simulink model "Sim_Modell_v5"  (R2021b)
settings: Solver=daessc  StartTime=0.0  StopTime=100  RelTol=1e-3
undefined symbols (not defined in the file): neg, pos, sigbuilder_block
libraries: fl_lib x25, nesl_utility x17, ee_lib x1, simulink x1
settings Model: Creator=lisa-  LastModifiedBy=felix

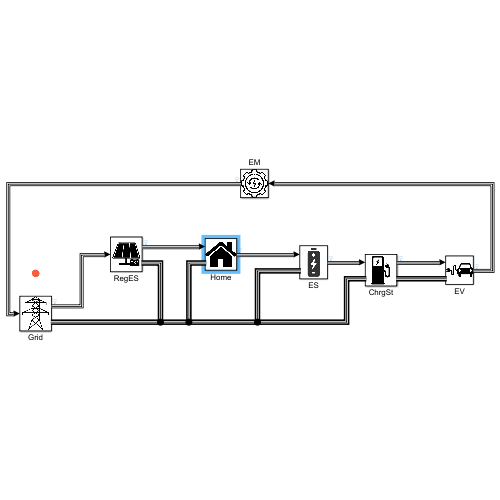
[thumbnail: Simulink's stored preview of the top-level diagram]
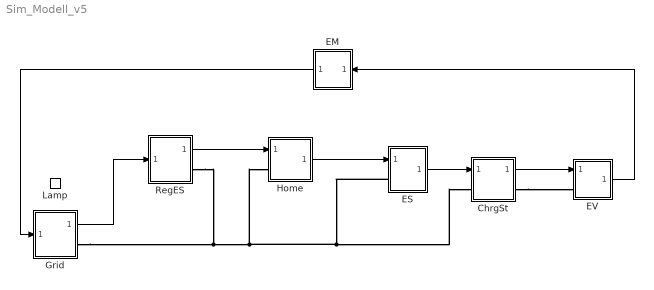
== system Sim_Modell_v5 ==
  ChrgSt : Subsystem
      settings: PortSchema="{\"entries\":[{\"content\":{\"sides\":[{\"content\":{\"connectorIds\":[]},\"type\":\"ConnectorPlacement.EquallySpacedRectSide\",\"uuid\":\"b41e38a9-5af4-4fc3-8362-b0a2c9ea7f09\"},{\"content\":{\"connectorIds\":[],\"side\":\"RIGHT\"},\"type\":\"ConnectorPlacement.EquallySpacedRectSide\",\"uuid\":\"3d2284f1-ff92-4301-996c-df10035f8991\"},{\"content\":{\"connectorIds\":[\"In1\",\"LConn1\"],\"side\":\"TOP\"},\"type\":\"ConnectorPlacement.EquallySpacedRectSide\",\"uuid\":\"3c162699-1ee7-4b12-b844-90d345f681c2\"},{\"content\":{\"connectorIds\":[\"Out1\",\"RConn1\"],\"side\":\"BOTTOM\"},\"type\":\"ConnectorPlacement.EquallySpacedRectSide\",\"uuid\":\"c143c3a3-5e1b-42e8-ba00-2d87f1345ae6\"}]},\"type\":\"ConnectorPlacement.EquallySpacedConnector\",\"uuid\":\"20a307e0-46b7-49be-a325-e97621053049\"}],\"packageUris\":[\"http://schema.mathworks.com/mf0/Connector/R2020b\"],\"version\":\"1.0\"}"
      mask Display: image('D:\Felix\Studium HTW Dresden\8. Semester\Matlab\Bilder\ChrgSt_icon.png'); % Use "Edit Image" on toolstrip to change.
  EM : Subsystem
      mask Display: image('D:\Felix\Studium HTW Dresden\8. Semester\Matlab\Bilder\EM_icon.png'); % Use "Edit Image" on toolstrip to change.
  ES : Subsystem
      mask Display: image('D:\Felix\Studium HTW Dresden\8. Semester\Matlab\Bilder\ES_icon.png'); % Use "Edit Image" on toolstrip to change.
  EV : Subsystem
      mask Display: image('D:\Felix\Studium HTW Dresden\8. Semester\Matlab\Bilder\electric_car_icon.jpg'); % Use "Edit Image" on toolstrip to change.
  Grid : Subsystem
      mask Display: image('D:\Felix\Studium HTW Dresden\8. Semester\Matlab\Bilder\Grid_icon.webp'); % Use "Edit Image" on toolstrip to change.
  Home : Subsystem
      mask Display: image('D:\Felix\Studium HTW Dresden\8. Semester\Matlab\Bilder\Home_icon.png'); % Use "Edit Image" on toolstrip to change.
  Lamp : LampBlock  LabelPosition=Hide
  RegES : Subsystem
      mask Display: image('D:\Felix\Studium HTW Dresden\8. Semester\Matlab\Bilder\solar_storage_icon.png'); % Use "Edit Image" on toolstrip to change.
  wires:
  RegES/1(Out1) -> Home/1(In1)
  Grid/1(Out1) -> RegES/1(In1)
  ES/1(Out1) -> ChrgSt/1(In1)
  ChrgSt/1(Out1) -> EV/1(In1)
  EV/1(Out1) -> EM/1(In1)
  Home/1(Out1) -> ES/1(In1)
  EM/1(Out1) -> Grid/1(In1)
  connections:
  Grid/RConn1 -- RegES/RConn1 -- ES/LConn1 -- ChrgSt/LConn1 -- Home/LConn1
  ChrgSt/RConn1 -- EV/LConn1

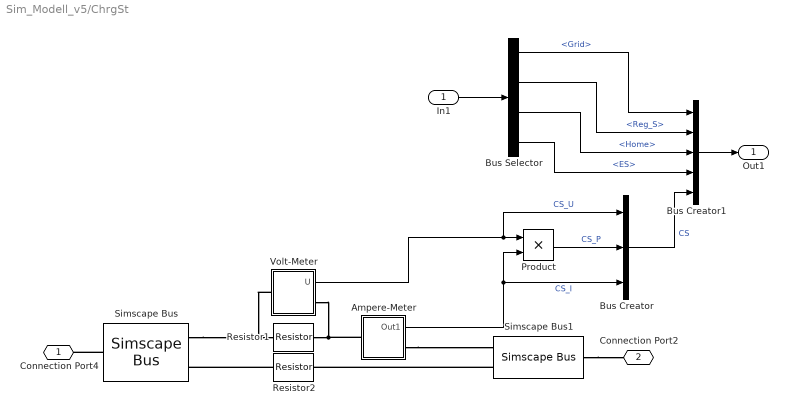
== system Sim_Modell_v5/ChrgSt ==
  In1 : Inport
  Ampere-Meter : Subsystem  mask{tc=0.01}
      mask prompts: tc "time constant"
      mask Display: image('D:\Felix\Studium HTW Dresden\8. Semester\Matlab\Bilder\ampere_icon.svg'); % Use "Edit Image" on toolstrip to change.
  Bus Creator : BusCreator  Inputs=3
  Bus Creator1 : BusCreator  Inputs=5
  Bus Selector : BusSelector  OutputSignals=Grid,Reg_S,Home,ES
  Product : Product
  Resistor1 : fl_lib/Electrical/Electrical Elements/Resistor  R=1 Ohm  i_specify=off  i_priority=None  i=0 A  i_nominal_specify=off  i_nominal_unit=A  i_nominal_value=1  v_specify=off  v_priority=None  v=0 V  v_nominal_specify=off  v_nominal_unit=V  v_nominal_value=1
  Resistor2 : fl_lib/Electrical/Electrical Elements/Resistor  R=1 Ohm  i_specify=off  i_priority=None  i=0 A  i_nominal_specify=off  i_nominal_unit=A  i_nominal_value=1  v_specify=off  v_priority=None  v=0 V  v_nominal_specify=off  v_nominal_unit=V  v_nominal_value=1
  Simscape Bus : SimscapeBus  HierarchyStrings=pos;neg
  Simscape Bus1 : SimscapeBus  HierarchyStrings=pos;neg
  Volt-Meter : Subsystem  mask{tc=0.01}
      mask prompts: tc "time constant"
      mask Display: image('D:\Felix\Studium HTW Dresden\8. Semester\Matlab\Bilder\volt_icon.svg'); % Use "Edit Image" on toolstrip to change.
  Connection Port4 : PMIOPort  Side=Left
  Connection Port2 : PMIOPort  Port=2  Side=Right
  Out1 : Outport
  wires:
  Volt-Meter/1(U) -> Bus Creator/1, Product/1  "CS_U"
  Ampere-Meter/1(Out1) -> Product/2, Bus Creator/3  "CS_I"
  Product/1 -> Bus Creator/2  "CS_P"
  In1/1 -> Bus Selector/1
  Bus Creator1/1 -> Out1/1
  Bus Selector/1 -> Bus Creator1/1  "<Grid>"
  Bus Selector/2 -> Bus Creator1/2  "<Reg_S>"
  Bus Selector/3 -> Bus Creator1/3  "<Home>"
  Bus Selector/4 -> Bus Creator1/4  "<ES>"
  Bus Creator/1 -> Bus Creator1/5  "CS"
  connections:
  Resistor1/RConn1 -- Volt-Meter/RConn1 -- Ampere-Meter/LConn1
  Simscape Bus/RConn1 -- Connection Port4/RConn1
  Simscape Bus1/RConn1 -- Connection Port2/RConn1
  Simscape Bus/LConn1 -- Volt-Meter/LConn1 -- Resistor1/LConn1
  Resistor2/RConn1 -- Simscape Bus/LConn2
  Ampere-Meter/RConn1 -- Simscape Bus1/LConn1
  Simscape Bus1/LConn2 -- Resistor2/LConn1

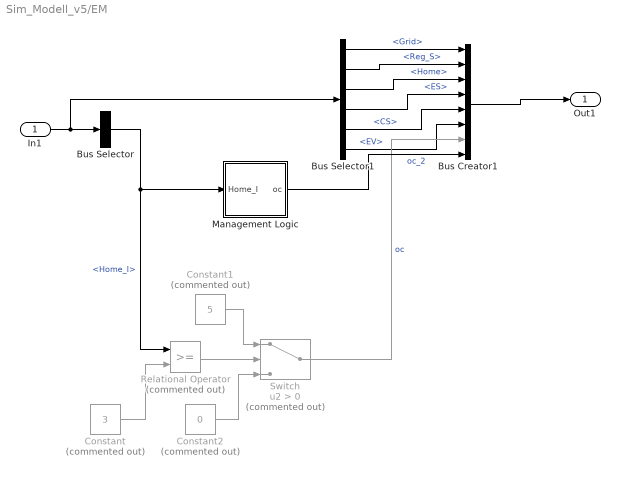
== system Sim_Modell_v5/EM ==
  In1 : Inport
  Bus Creator1 : BusCreator  Inputs=8
  Bus Selector : BusSelector  OutputSignals=Home.Home_I
  Bus Selector1 : BusSelector  OutputSignals=Grid,Reg_S,Home,ES,CS,EV
  Constant : Constant  Commented=on  Value=3
  Constant1 : Constant  Commented=on  Value=5
  Constant2 : Constant  Commented=on  Value=0
  Management Logic : Stateflow chart  TreatAsAtomicUnit=on
  Relational Operator : RelationalOperator  Commented=on  OutDataTypeStr=boolean  RndMeth=Simplest
  Switch : Switch  Commented=on  Criteria=u2 > Threshold
  Out1 : Outport
  wires:
  In1/1 -> Bus Selector1/1, Bus Selector/1
  Constant/1 -> Relational Operator/2
  Relational Operator/1 -> Switch/2
  Constant2/1 -> Switch/3
  Constant1/1 -> Switch/1
  Bus Selector1/3 -> Bus Creator1/3  "<Home>"
  Bus Selector1/1 -> Bus Creator1/1  "<Grid>"
  Bus Selector1/2 -> Bus Creator1/2  "<Reg_S>"
  Bus Selector1/4 -> Bus Creator1/4  "<ES>"
  Bus Selector1/5 -> Bus Creator1/5  "<CS>"
  Bus Selector1/6 -> Bus Creator1/6  "<EV>"
  Bus Creator1/1 -> Out1/1
  Bus Selector/1 -> Management Logic/1(Home_I), Relational Operator/1  "<Home_I>"
  Switch/1 -> Bus Creator1/7  "oc"
  Management Logic/1(oc) -> Bus Creator1/8  "oc_2"

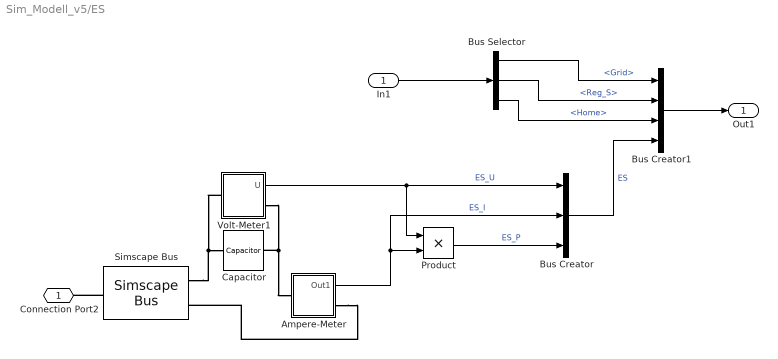
== system Sim_Modell_v5/ES ==
  In1 : Inport
  Ampere-Meter : Subsystem  mask{tc=0.01}
      mask prompts: tc "time constant"
      mask Display: image('D:\Felix\Studium HTW Dresden\8. Semester\Matlab\Bilder\ampere_icon.svg'); % Use "Edit Image" on toolstrip to change.
  Bus Creator : BusCreator  Inputs=3
  Bus Creator1 : BusCreator  Inputs=4
  Bus Selector : BusSelector  OutputSignals=Grid,Reg_S,Home
  Capacitor : fl_lib/Electrical/Electrical Elements/Capacitor  c=1e-6 F  r=1e-6 Ohm  g=0 1/Ohm  i_specify=off  i_priority=None  i=0 A  i_nominal_specify=off  i_nominal_unit=A  i_nominal_value=1  v_specify=off  v_priority=None  v=0 V  v_nominal_specify=off  v_nominal_unit=V  v_nominal_value=1  vc_specify=off  vc_priority=High  vc=0 V  vc_nominal_specify=off  vc_nominal_unit=V  vc_nominal_value=1
  Product : Product
  Simscape Bus : SimscapeBus  HierarchyStrings=pos;neg
  Volt-Meter1 : Subsystem  mask{tc=0.01}
      mask prompts: tc "time constant"
      mask Display: image('D:\Felix\Studium HTW Dresden\8. Semester\Matlab\Bilder\volt_icon.svg'); % Use "Edit Image" on toolstrip to change.
  Connection Port2 : PMIOPort  Side=Left
  Out1 : Outport
  wires:
  Volt-Meter1/1(U) -> Bus Creator/1, Product/1  "ES_U"
  Ampere-Meter/1(Out1) -> Bus Creator/2, Product/2  "ES_I"
  Product/1 -> Bus Creator/3  "ES_P"
  In1/1 -> Bus Selector/1
  Bus Selector/1 -> Bus Creator1/1  "<Grid>"
  Bus Selector/2 -> Bus Creator1/2  "<Reg_S>"
  Bus Selector/3 -> Bus Creator1/3  "<Home>"
  Bus Creator/1 -> Bus Creator1/4  "ES"
  Bus Creator1/1 -> Out1/1
  connections:
  Simscape Bus/LConn1 -- Volt-Meter1/LConn1 -- Capacitor/LConn1
  Volt-Meter1/RConn1 -- Ampere-Meter/LConn1 -- Capacitor/RConn1
  Simscape Bus/RConn1 -- Connection Port2/RConn1
  Ampere-Meter/RConn1 -- Simscape Bus/LConn2

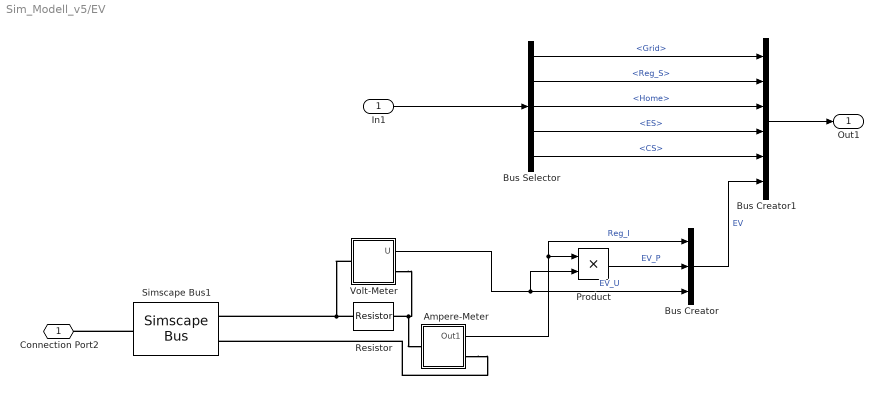
== system Sim_Modell_v5/EV ==
  In1 : Inport
  Ampere-Meter : Subsystem  mask{tc=0.01}
      mask prompts: tc "time constant"
      mask Display: image('D:\Felix\Studium HTW Dresden\8. Semester\Matlab\Bilder\ampere_icon.svg'); % Use "Edit Image" on toolstrip to change.
  Bus Creator : BusCreator  Inputs=3
  Bus Creator1 : BusCreator  Inputs=6
  Bus Selector : BusSelector  OutputSignals=Grid,Reg_S,Home,ES,CS
  Product : Product
  Resistor : fl_lib/Electrical/Electrical Elements/Resistor  R=1 Ohm  i_specify=off  i_priority=None  i=0 A  i_nominal_specify=off  i_nominal_unit=A  i_nominal_value=1  v_specify=off  v_priority=None  v=0 V  v_nominal_specify=off  v_nominal_unit=V  v_nominal_value=1
  Simscape Bus1 : SimscapeBus  HierarchyStrings=pos;neg
  Volt-Meter : Subsystem  mask{tc=0.01}
      mask prompts: tc "time constant"
      mask Display: image('D:\Felix\Studium HTW Dresden\8. Semester\Matlab\Bilder\volt_icon.svg'); % Use "Edit Image" on toolstrip to change.
  Connection Port2 : PMIOPort  Side=Left
  Out1 : Outport
  wires:
  Volt-Meter/1(U) -> Product/2, Bus Creator/3  "EV_U"
  Product/1 -> Bus Creator/2  "EV_P"
  In1/1 -> Bus Selector/1
  Bus Creator/1 -> Bus Creator1/6  "EV"
  Bus Selector/5 -> Bus Creator1/5  "<CS>"
  Bus Selector/4 -> Bus Creator1/4  "<ES>"
  Bus Selector/3 -> Bus Creator1/3  "<Home>"
  Bus Selector/2 -> Bus Creator1/2  "<Reg_S>"
  Bus Selector/1 -> Bus Creator1/1  "<Grid>"
  Bus Creator1/1 -> Out1/1
  Ampere-Meter/1(Out1) -> Product/1, Bus Creator/1  "Reg_I"
  connections:
  Simscape Bus1/RConn1 -- Connection Port2/RConn1
  Resistor/RConn1 -- Volt-Meter/RConn1 -- Ampere-Meter/LConn1
  Resistor/LConn1 -- Volt-Meter/LConn1 -- Simscape Bus1/LConn1
  Ampere-Meter/RConn1 -- Simscape Bus1/LConn2

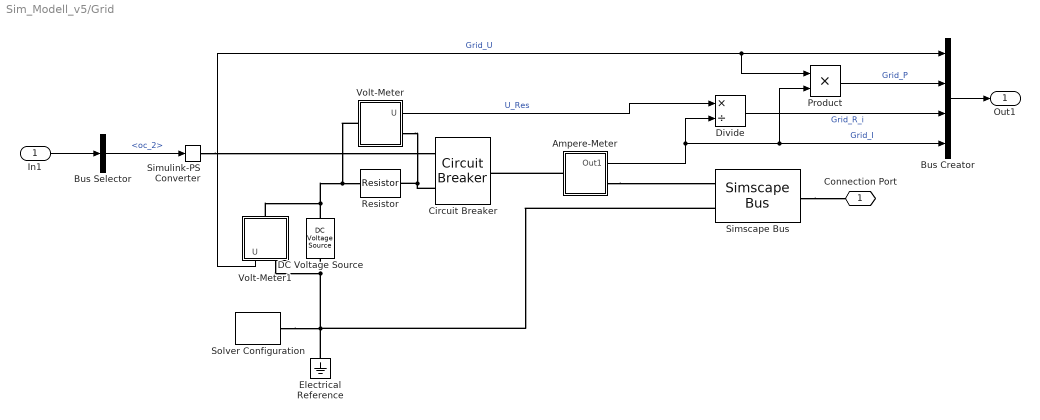
== system Sim_Modell_v5/Grid ==
  In1 : Inport
  Ampere-Meter : Subsystem  mask{tc=0.01}
      mask prompts: tc "time constant"
      mask Display: image('D:\Felix\Studium HTW Dresden\8. Semester\Matlab\Bilder\ampere_icon.svg'); % Use "Edit Image" on toolstrip to change.
  Bus Creator : BusCreator  Inputs=4
  Bus Selector : BusSelector  OutputSignals=oc_2
  Circuit Breaker : ee_lib/Switches & Breakers/Circuit Breaker  R_closed=0.001 Ohm  G_open=1e-6 1/Ohm  threshold=1 V  offset_for_on=1 V
      settings: SourceProductBaseCode=PS  InternalSimscapePortConfiguration="{\"Bottom\":[],\"Left\":[{\"id\":\"vT\",\"label\":\"vT\",\"type\":\"input\"},{\"id\":\"p1\",\"label\":\"\",\"type\":\"foundation.electrical.electrical\"}],\"Right\":[{\"id\":\"p2\",\"label\":\"\",\"type\":\"foundation.electrical.electrical\"}],\"Top\":[]}"
  DC Voltage Source : fl_lib/Electrical/Electrical Sources/DC Voltage Source  v0=10 V
  Divide : Product  Inputs=*/
  Electrical Reference : fl_lib/Electrical/Electrical Elements/Electrical Reference
  Product : Product
  Resistor : fl_lib/Electrical/Electrical Elements/Resistor  R=1 Ohm  i_specify=off  i_priority=None  i=0 A  i_nominal_specify=off  i_nominal_unit=A  i_nominal_value=1  v_specify=off  v_priority=None  v=0 V  v_nominal_specify=off  v_nominal_unit=V  v_nominal_value=1
  Simscape Bus : SimscapeBus  HierarchyStrings=pos;neg
  Simulink-PS Converter : nesl_utility/Simulink-PS Converter  PhysicalDomain=network_engine_domain  SubClassName=ps_input  LeftPortType=input  RightPortType=output  PseudoPeriodic=off  Frequencies=[]  NoiseDistribution=none  NoiseParameters=[]  Unit=V  AffineConversion=off  FilteringAndDerivatives=provide  SimscapeFilterOrder=1  InputFilterTimeConstant=0.001  UdotUserProvided=0
      settings: SourceProductBaseCode=PW,SS
  Solver Configuration : nesl_utility/Solver Configuration  PhysicalDomain=network_engine_domain  SubClassName=solver  LeftPortType=input  RightPortType=generic  Tones=[]  Harmonics=[]  SimulateNoise=off  Profile=off  UseLocalSampling=off  EnableSwitchedLinearOptims=on  FrequencyDomain=off  UseCCode=off  RelTol=0.001  AbsTol=1e-06  MinStep=1e-09  ToWorkspace=off  RevertToSquareIcSolve=off  NumHomotopyIterations=100  PhasorMode=off  PhasorModeNumHarmonics=1  DoDC=off  ResidualTolerance=1e-09  UseLocalSolver=off  LocalSolverChoice=NE_BACKWARD_EULER_ADVANCER  LocalSolverSampleTime=0.001  DoFixedCost=off  MaxNonlinIter=3  MaxModeIter=2  ComputeImpulses=off  ImpulseIterations=2  LinearAlgebra=auto  EquationFormulation=NE_TIME_EF  DelaysMemoryBudget=1024  AutomaticFiltering=on  FilteringTimeConstant=0.001  PartitionStorageMethod=AS_NEEDED  PartitionMemoryBudget=1024  PartitionMethod=ROBUST
      settings: SourceProductBaseCode=PW,SS
  Volt-Meter : Subsystem  mask{tc=0.01}
      mask prompts: tc "time constant"
      mask Display: image('D:\Felix\Studium HTW Dresden\8. Semester\Matlab\Bilder\volt_icon.svg'); % Use "Edit Image" on toolstrip to change.
  Volt-Meter1 : Subsystem  mask{tc=0.01}
      mask prompts: tc "time constant"
      mask Display: image('D:\Felix\Studium HTW Dresden\8. Semester\Matlab\Bilder\volt_icon.svg'); % Use "Edit Image" on toolstrip to change.
  Connection Port : PMIOPort  Side=Right
  Out1 : Outport
  wires:
  Bus Creator/1 -> Out1/1
  Volt-Meter/1(U) -> Divide/1  "U_Res"
  Volt-Meter1/1(U) -> Product/1, Bus Creator/1  "Grid_U"
  Ampere-Meter/1(Out1) -> Divide/2, Product/2, Bus Creator/4  "Grid_I"
  Divide/1 -> Bus Creator/3  "Grid_R_i"
  Product/1 -> Bus Creator/2  "Grid_P"
  Bus Selector/1 -> Simulink-PS Converter/1  "<oc_2>"
  In1/1 -> Bus Selector/1
  connections:
  Solver Configuration/RConn1 -- Simscape Bus/LConn2 -- Electrical Reference/LConn1 -- Volt-Meter1/RConn1 -- DC Voltage Source/RConn1
  Simscape Bus/RConn1 -- Connection Port/RConn1
  DC Voltage Source/LConn1 -- Volt-Meter1/LConn1 -- Volt-Meter/LConn1 -- Resistor/LConn1
  Ampere-Meter/LConn1 -- Circuit Breaker/RConn1
  Ampere-Meter/RConn1 -- Simscape Bus/LConn1
  Circuit Breaker/LConn2 -- Volt-Meter/RConn1 -- Resistor/RConn1
  Simulink-PS Converter/RConn1 -- Circuit Breaker/LConn1

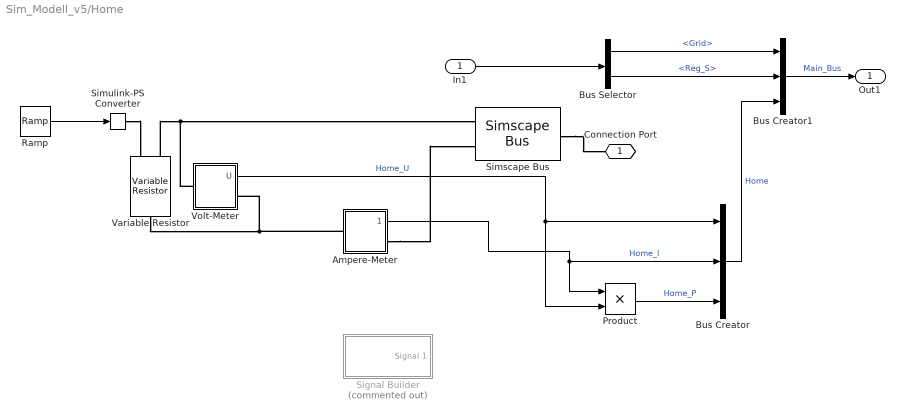
== system Sim_Modell_v5/Home ==
  In1 : Inport
  Ampere-Meter : Subsystem  mask{tc=0.01}
      mask prompts: tc "time constant"
      mask Display: image('D:\Felix\Studium HTW Dresden\8. Semester\Matlab\Bilder\ampere_icon.svg'); % Use "Edit Image" on toolstrip to change.
  Bus Creator : BusCreator  Inputs=3
  Bus Creator1 : BusCreator  Inputs=3
  Bus Selector : BusSelector  OutputSignals=Grid,Reg_S
  Product : Product
  Ramp : simulink/Sources/Ramp  slope=-2.5  start=0  InitialOutput=100
  Signal Builder : Subsystem  Tag=STV Subsys  Commented=on  LoadFcn=sigbuilder_block('load');  StartFcn=sigbuilder_block('start');  StopFcn=sigbuilder_block('stop');  ClipboardFcn=sigbuilder_block('clipboard');  mask(Sigbuilder block){tuvar=[0:10]}
      mask help: Simulink:masks:SigbuilderBlock_MD
      mask init:
      | if ~strcmp(get_param(bdroot(gcbh),'SimulationStatus'),'stopped') tuvar = sigbuilder_block('maskInit'); end
      settings: CopyFcn=sigbuilder_block('copy');  DeleteFcn=sigbuilder_block('delete');  ModelCloseFcn=sigbuilder_block('modelClose');  PreSaveFcn=sigbuilder_block('preSave');  PauseFcn=sigbuilder_block('pause');  ContinueFcn=sigbuilder_block('continue');  NameChangeFcn=sigbuilder_block('namechange');  OpenFcn=sigbuilder_block('open',[373.8 119.4 550.8 400.2 ]);  CloseFcn=sigbuilder_block('close');
      mask Display: plot(0, 0, 100, 100,[2, 2, 32, 32, 2], [68, 8, 8, 68, 68],[32, 2], [38, 38], [32, 19, 2],[53, 60, 44], [32, 17, 17, 2],[16, 16, 31, 31]);txt = getActiveGroup(gcbh);text(2, 100, txt,'verticalAlignment', 'top');
  Simscape Bus : SimscapeBus  HierarchyStrings=pos;neg
  Simulink-PS Converter : nesl_utility/Simulink-PS Converter  PhysicalDomain=network_engine_domain  SubClassName=ps_input  LeftPortType=input  RightPortType=output  PseudoPeriodic=off  Frequencies=[]  NoiseDistribution=none  NoiseParameters=[]  Unit=1  AffineConversion=off  FilteringAndDerivatives=provide  SimscapeFilterOrder=1  InputFilterTimeConstant=0.001  UdotUserProvided=0
      settings: SourceProductBaseCode=PW,SS
  Variable Resistor : fl_lib/Electrical/Electrical Elements/Variable Resistor  Rmin=0 Ohm  i_specify=off  i_priority=None  i=0 A  i_nominal_specify=off  i_nominal_unit=A  i_nominal_value=1  v_specify=off  v_priority=None  v=0 V  v_nominal_specify=off  v_nominal_unit=V  v_nominal_value=1
  Volt-Meter : Subsystem  mask{tc=0.01}
      mask prompts: tc "time constant"
      mask Display: image('D:\Felix\Studium HTW Dresden\8. Semester\Matlab\Bilder\volt_icon.svg'); % Use "Edit Image" on toolstrip to change.
  Connection Port : PMIOPort  Side=Left
  Out1 : Outport
  wires:
  Ramp/1 -> Simulink-PS Converter/1
  Volt-Meter/1(U) -> Product/2, Bus Creator/1  "Home_U"
  Product/1 -> Bus Creator/3  "Home_P"
  In1/1 -> Bus Selector/1
  Bus Creator/1 -> Bus Creator1/3  "Home"
  Bus Selector/1 -> Bus Creator1/1  "<Grid>"
  Bus Selector/2 -> Bus Creator1/2  "<Reg_S>"
  Bus Creator1/1 -> Out1/1  "Main_Bus"
  Ampere-Meter/1(Home_I) -> Bus Creator/2, Product/1  "Home_I"
  connections:
  Simulink-PS Converter/RConn1 -- Variable Resistor/LConn1
  Variable Resistor/LConn2 -- Simscape Bus/LConn1 -- Volt-Meter/LConn1
  Simscape Bus/RConn1 -- Connection Port/RConn1
  Variable Resistor/RConn1 -- Ampere-Meter/LConn1 -- Volt-Meter/RConn1
  Ampere-Meter/RConn1 -- Simscape Bus/LConn2

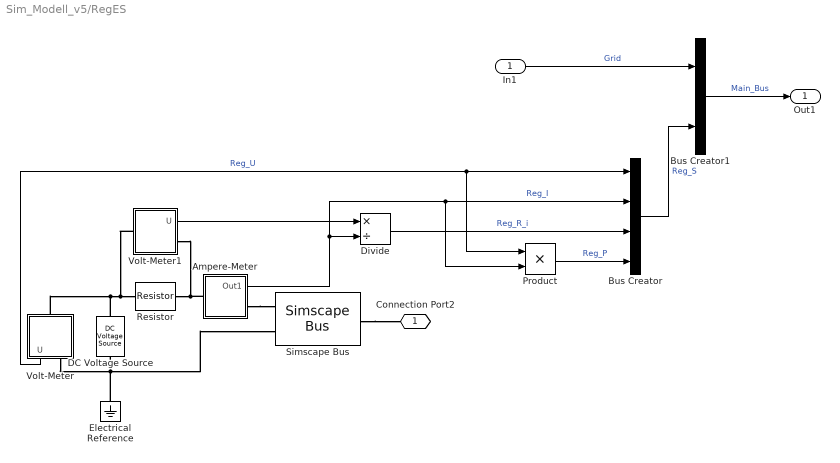
== system Sim_Modell_v5/RegES ==
  In1 : Inport
  Ampere-Meter : Subsystem  mask{tc=0.01}
      mask prompts: tc "time constant"
      mask Display: image('D:\Felix\Studium HTW Dresden\8. Semester\Matlab\Bilder\ampere_icon.svg'); % Use "Edit Image" on toolstrip to change.
  Bus Creator : BusCreator  Inputs=4
  Bus Creator1 : BusCreator  Inputs=2
  DC Voltage Source : fl_lib/Electrical/Electrical Sources/DC Voltage Source  v0=5 V
  Divide : Product  Inputs=*/
  Electrical Reference : fl_lib/Electrical/Electrical Elements/Electrical Reference
  Product : Product
  Resistor : fl_lib/Electrical/Electrical Elements/Resistor  R=1 Ohm  i_specify=off  i_priority=None  i=0 A  i_nominal_specify=off  i_nominal_unit=A  i_nominal_value=1  v_specify=off  v_priority=None  v=0 V  v_nominal_specify=off  v_nominal_unit=V  v_nominal_value=1
  Simscape Bus : SimscapeBus  HierarchyStrings=pos;neg
  Volt-Meter : Subsystem  mask{tc=0.01}
      mask prompts: tc "time constant"
      mask Display: image('D:\Felix\Studium HTW Dresden\8. Semester\Matlab\Bilder\volt_icon.svg'); % Use "Edit Image" on toolstrip to change.
  Volt-Meter1 : Subsystem  mask{tc=0.01}
      mask prompts: tc "time constant"
      mask Display: image('D:\Felix\Studium HTW Dresden\8. Semester\Matlab\Bilder\volt_icon.svg'); % Use "Edit Image" on toolstrip to change.
  Connection Port2 : PMIOPort  Side=Right
  Out1 : Outport
  wires:
  Volt-Meter/1(U) -> Product/1, Bus Creator/1  "Reg_U"
  Ampere-Meter/1(Out1) -> Product/2, Bus Creator/2, Divide/2  "Reg_I"
  Divide/1 -> Bus Creator/3  "Reg_R_i"
  Product/1 -> Bus Creator/4  "Reg_P"
  In1/1 -> Bus Creator1/1  "Grid"
  Bus Creator/1 -> Bus Creator1/2  "Reg_S"
  Bus Creator1/1 -> Out1/1  "Main_Bus"
  Volt-Meter1/1(U) -> Divide/1
  connections:
  Electrical Reference/LConn1 -- Volt-Meter/RConn1 -- Simscape Bus/LConn2 -- DC Voltage Source/RConn1
  Simscape Bus/RConn1 -- Connection Port2/RConn1
  DC Voltage Source/LConn1 -- Volt-Meter/LConn1 -- Volt-Meter1/LConn1 -- Resistor/LConn1
  Resistor/RConn1 -- Ampere-Meter/LConn1 -- Volt-Meter1/RConn1
  Ampere-Meter/RConn1 -- Simscape Bus/LConn1

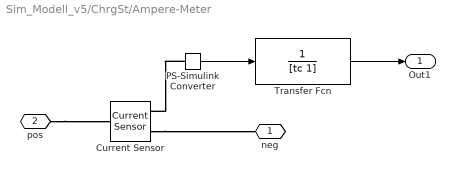
== system Sim_Modell_v5/ChrgSt/Ampere-Meter ==
  Current Sensor : fl_lib/Electrical/Electrical Sensors/Current Sensor
  PS-Simulink Converter : nesl_utility/PS-Simulink Converter  PhysicalDomain=network_engine_domain  SubClassName=ps_output  LeftPortType=input  RightPortType=output  PseudoPeriodic=off  Frequencies=[]  Unit=inherit  AffineConversion=on
      settings: SourceProductBaseCode=PW,SS
  Transfer Fcn : TransferFcn  Numerator=1  Denominator=[tc 1]
  neg : PMIOPort  Side=Right
  pos : PMIOPort  Port=2  Side=Left
  Out1 : Outport
  wires:
  PS-Simulink Converter/1 -> Transfer Fcn/1
  Transfer Fcn/1 -> Out1/1
  connections:
  PS-Simulink Converter/LConn1 -- Current Sensor/RConn1
  Current Sensor/RConn2 -- neg/RConn1
  pos/RConn1 -- Current Sensor/LConn1

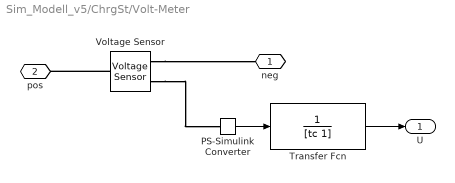
== system Sim_Modell_v5/ChrgSt/Volt-Meter ==
  PS-Simulink Converter : nesl_utility/PS-Simulink Converter  PhysicalDomain=network_engine_domain  SubClassName=ps_output  LeftPortType=input  RightPortType=output  PseudoPeriodic=off  Frequencies=[]  Unit=inherit  AffineConversion=on
      settings: SourceProductBaseCode=PW,SS
  Transfer Fcn : TransferFcn  Numerator=1  Denominator=[tc 1]
  Voltage Sensor : fl_lib/Electrical/Electrical Sensors/Voltage Sensor
  neg : PMIOPort  Side=Right
  pos : PMIOPort  Port=2  Side=Left
  U : Outport
  wires:
  PS-Simulink Converter/1 -> Transfer Fcn/1
  Transfer Fcn/1 -> U/1
  connections:
  Voltage Sensor/RConn1 -- PS-Simulink Converter/LConn1
  Voltage Sensor/RConn2 -- neg/RConn1
  Voltage Sensor/LConn1 -- pos/RConn1

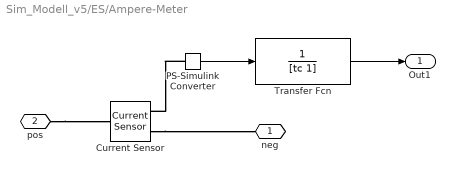
== system Sim_Modell_v5/ES/Ampere-Meter ==
  Current Sensor : fl_lib/Electrical/Electrical Sensors/Current Sensor
  PS-Simulink Converter : nesl_utility/PS-Simulink Converter  PhysicalDomain=network_engine_domain  SubClassName=ps_output  LeftPortType=input  RightPortType=output  PseudoPeriodic=off  Frequencies=[]  Unit=inherit  AffineConversion=on
      settings: SourceProductBaseCode=PW,SS
  Transfer Fcn : TransferFcn  Numerator=1  Denominator=[tc 1]
  neg : PMIOPort  Side=Right
  pos : PMIOPort  Port=2  Side=Left
  Out1 : Outport
  wires:
  PS-Simulink Converter/1 -> Transfer Fcn/1
  Transfer Fcn/1 -> Out1/1
  connections:
  PS-Simulink Converter/LConn1 -- Current Sensor/RConn1
  Current Sensor/RConn2 -- neg/RConn1
  pos/RConn1 -- Current Sensor/LConn1

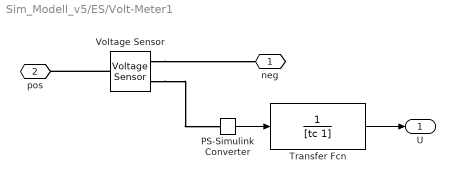
== system Sim_Modell_v5/ES/Volt-Meter1 ==
  PS-Simulink Converter : nesl_utility/PS-Simulink Converter  PhysicalDomain=network_engine_domain  SubClassName=ps_output  LeftPortType=input  RightPortType=output  PseudoPeriodic=off  Frequencies=[]  Unit=inherit  AffineConversion=on
      settings: SourceProductBaseCode=PW,SS
  Transfer Fcn : TransferFcn  Numerator=1  Denominator=[tc 1]
  Voltage Sensor : fl_lib/Electrical/Electrical Sensors/Voltage Sensor
  neg : PMIOPort  Side=Right
  pos : PMIOPort  Port=2  Side=Left
  U : Outport
  wires:
  PS-Simulink Converter/1 -> Transfer Fcn/1
  Transfer Fcn/1 -> U/1
  connections:
  Voltage Sensor/RConn1 -- PS-Simulink Converter/LConn1
  Voltage Sensor/RConn2 -- neg/RConn1
  Voltage Sensor/LConn1 -- pos/RConn1

== system Sim_Modell_v5/EV/Ampere-Meter ==
  Current Sensor : fl_lib/Electrical/Electrical Sensors/Current Sensor
  PS-Simulink Converter : nesl_utility/PS-Simulink Converter  PhysicalDomain=network_engine_domain  SubClassName=ps_output  LeftPortType=input  RightPortType=output  PseudoPeriodic=off  Frequencies=[]  Unit=inherit  AffineConversion=on
      settings: SourceProductBaseCode=PW,SS
  Transfer Fcn : TransferFcn  Numerator=1  Denominator=[tc 1]
  neg : PMIOPort  Side=Right
  pos : PMIOPort  Port=2  Side=Left
  Out1 : Outport
  wires:
  PS-Simulink Converter/1 -> Transfer Fcn/1
  Transfer Fcn/1 -> Out1/1
  connections:
  PS-Simulink Converter/LConn1 -- Current Sensor/RConn1
  Current Sensor/RConn2 -- neg/RConn1
  pos/RConn1 -- Current Sensor/LConn1

== system Sim_Modell_v5/EV/Volt-Meter ==
  PS-Simulink Converter : nesl_utility/PS-Simulink Converter  PhysicalDomain=network_engine_domain  SubClassName=ps_output  LeftPortType=input  RightPortType=output  PseudoPeriodic=off  Frequencies=[]  Unit=inherit  AffineConversion=on
      settings: SourceProductBaseCode=PW,SS
  Transfer Fcn : TransferFcn  Numerator=1  Denominator=[tc 1]
  Voltage Sensor : fl_lib/Electrical/Electrical Sensors/Voltage Sensor
  neg : PMIOPort  Side=Right
  pos : PMIOPort  Port=2  Side=Left
  U : Outport
  wires:
  PS-Simulink Converter/1 -> Transfer Fcn/1
  Transfer Fcn/1 -> U/1
  connections:
  Voltage Sensor/RConn1 -- PS-Simulink Converter/LConn1
  Voltage Sensor/RConn2 -- neg/RConn1
  Voltage Sensor/LConn1 -- pos/RConn1

== system Sim_Modell_v5/Grid/Ampere-Meter ==
  Current Sensor : fl_lib/Electrical/Electrical Sensors/Current Sensor
  PS-Simulink Converter : nesl_utility/PS-Simulink Converter  PhysicalDomain=network_engine_domain  SubClassName=ps_output  LeftPortType=input  RightPortType=output  PseudoPeriodic=off  Frequencies=[]  Unit=inherit  AffineConversion=on
      settings: SourceProductBaseCode=PW,SS
  Transfer Fcn : TransferFcn  Numerator=1  Denominator=[tc 1]
  neg : PMIOPort  Side=Right
  pos : PMIOPort  Port=2  Side=Left
  Out1 : Outport
  wires:
  PS-Simulink Converter/1 -> Transfer Fcn/1
  Transfer Fcn/1 -> Out1/1
  connections:
  PS-Simulink Converter/LConn1 -- Current Sensor/RConn1
  Current Sensor/RConn2 -- neg/RConn1
  pos/RConn1 -- Current Sensor/LConn1

== system Sim_Modell_v5/Grid/Volt-Meter ==
  PS-Simulink Converter : nesl_utility/PS-Simulink Converter  PhysicalDomain=network_engine_domain  SubClassName=ps_output  LeftPortType=input  RightPortType=output  PseudoPeriodic=off  Frequencies=[]  Unit=inherit  AffineConversion=on
      settings: SourceProductBaseCode=PW,SS
  Transfer Fcn : TransferFcn  Numerator=1  Denominator=[tc 1]
  Voltage Sensor : fl_lib/Electrical/Electrical Sensors/Voltage Sensor
  neg : PMIOPort  Side=Right
  pos : PMIOPort  Port=2  Side=Left
  U : Outport
  wires:
  PS-Simulink Converter/1 -> Transfer Fcn/1
  Transfer Fcn/1 -> U/1
  connections:
  Voltage Sensor/RConn1 -- PS-Simulink Converter/LConn1
  Voltage Sensor/RConn2 -- neg/RConn1
  Voltage Sensor/LConn1 -- pos/RConn1

== system Sim_Modell_v5/Grid/Volt-Meter1 ==
  PS-Simulink Converter : nesl_utility/PS-Simulink Converter  PhysicalDomain=network_engine_domain  SubClassName=ps_output  LeftPortType=input  RightPortType=output  PseudoPeriodic=off  Frequencies=[]  Unit=inherit  AffineConversion=on
      settings: SourceProductBaseCode=PW,SS
  Transfer Fcn : TransferFcn  Numerator=1  Denominator=[tc 1]
  Voltage Sensor : fl_lib/Electrical/Electrical Sensors/Voltage Sensor
  neg : PMIOPort  Side=Right
  pos : PMIOPort  Port=2  Side=Left
  U : Outport
  wires:
  PS-Simulink Converter/1 -> Transfer Fcn/1
  Transfer Fcn/1 -> U/1
  connections:
  Voltage Sensor/RConn1 -- PS-Simulink Converter/LConn1
  Voltage Sensor/RConn2 -- neg/RConn1
  Voltage Sensor/LConn1 -- pos/RConn1

== system Sim_Modell_v5/Home/Ampere-Meter ==
  Current Sensor : fl_lib/Electrical/Electrical Sensors/Current Sensor
  PS-Simulink Converter : nesl_utility/PS-Simulink Converter  PhysicalDomain=network_engine_domain  SubClassName=ps_output  LeftPortType=input  RightPortType=output  PseudoPeriodic=off  Frequencies=[]  Unit=inherit  AffineConversion=on
      settings: SourceProductBaseCode=PW,SS
  Transfer Fcn : TransferFcn  Numerator=1  Denominator=[tc 1]
  neg : PMIOPort  Side=Right
  pos : PMIOPort  Port=2  Side=Left
  Home_I : Outport
  wires:
  PS-Simulink Converter/1 -> Transfer Fcn/1  "Home_I_1"
  Transfer Fcn/1 -> Home_I/1  "Home_I"
  connections:
  PS-Simulink Converter/LConn1 -- Current Sensor/RConn1
  Current Sensor/RConn2 -- neg/RConn1
  pos/RConn1 -- Current Sensor/LConn1

== system Sim_Modell_v5/Home/Signal Builder ==
  Demux : Demux  Tag=STV Demux  Outputs=1
      settings: DisplayOption=none
  FromWs : FromWorkspace  Tag=STV FromWs  VariableName=tuvar
      SigBuilderData=|
      | common.afterFinalStr = 'Extrapolate'
      | common.sampleTime = 0
      | dataSet.timeRange = [0 10]
      | dataSet.name = 'Group 1'
      | sbobj.Groups.Name = 'Group 1'
      | sbobj.Groups.Signals.Name = 'Signal 1'
      | sbobj.Groups.Signals.XData = [0 4 4 6 6 10]
      | sbobj.Groups.Signals.YData = [0 0 1 1 0 0]
  Signal 1 : Outport  Tag=STV Outport
  wires:
  Demux/1 -> Signal 1/1
  FromWs/1 -> Demux/1

== system Sim_Modell_v5/Home/Volt-Meter ==
  PS-Simulink Converter : nesl_utility/PS-Simulink Converter  PhysicalDomain=network_engine_domain  SubClassName=ps_output  LeftPortType=input  RightPortType=output  PseudoPeriodic=off  Frequencies=[]  Unit=inherit  AffineConversion=on
      settings: SourceProductBaseCode=PW,SS
  Transfer Fcn : TransferFcn  Numerator=1  Denominator=[tc 1]
  Voltage Sensor : fl_lib/Electrical/Electrical Sensors/Voltage Sensor
  neg : PMIOPort  Side=Right
  pos : PMIOPort  Port=2  Side=Left
  U : Outport
  wires:
  PS-Simulink Converter/1 -> Transfer Fcn/1
  Transfer Fcn/1 -> U/1
  connections:
  Voltage Sensor/RConn1 -- PS-Simulink Converter/LConn1
  Voltage Sensor/RConn2 -- neg/RConn1
  Voltage Sensor/LConn1 -- pos/RConn1

== system Sim_Modell_v5/RegES/Ampere-Meter ==
  Current Sensor : fl_lib/Electrical/Electrical Sensors/Current Sensor
  PS-Simulink Converter : nesl_utility/PS-Simulink Converter  PhysicalDomain=network_engine_domain  SubClassName=ps_output  LeftPortType=input  RightPortType=output  PseudoPeriodic=off  Frequencies=[]  Unit=inherit  AffineConversion=on
      settings: SourceProductBaseCode=PW,SS
  Transfer Fcn : TransferFcn  Numerator=1  Denominator=[tc 1]
  neg : PMIOPort  Side=Right
  pos : PMIOPort  Port=2  Side=Left
  Out1 : Outport
  wires:
  PS-Simulink Converter/1 -> Transfer Fcn/1
  Transfer Fcn/1 -> Out1/1
  connections:
  PS-Simulink Converter/LConn1 -- Current Sensor/RConn1
  Current Sensor/RConn2 -- neg/RConn1
  pos/RConn1 -- Current Sensor/LConn1

== system Sim_Modell_v5/RegES/Volt-Meter ==
  PS-Simulink Converter : nesl_utility/PS-Simulink Converter  PhysicalDomain=network_engine_domain  SubClassName=ps_output  LeftPortType=input  RightPortType=output  PseudoPeriodic=off  Frequencies=[]  Unit=inherit  AffineConversion=on
      settings: SourceProductBaseCode=PW,SS
  Transfer Fcn : TransferFcn  Numerator=1  Denominator=[tc 1]
  Voltage Sensor : fl_lib/Electrical/Electrical Sensors/Voltage Sensor
  neg : PMIOPort  Side=Right
  pos : PMIOPort  Port=2  Side=Left
  U : Outport
  wires:
  PS-Simulink Converter/1 -> Transfer Fcn/1
  Transfer Fcn/1 -> U/1
  connections:
  Voltage Sensor/RConn1 -- PS-Simulink Converter/LConn1
  Voltage Sensor/RConn2 -- neg/RConn1
  Voltage Sensor/LConn1 -- pos/RConn1

== system Sim_Modell_v5/RegES/Volt-Meter1 ==
  PS-Simulink Converter : nesl_utility/PS-Simulink Converter  PhysicalDomain=network_engine_domain  SubClassName=ps_output  LeftPortType=input  RightPortType=output  PseudoPeriodic=off  Frequencies=[]  Unit=inherit  AffineConversion=on
      settings: SourceProductBaseCode=PW,SS
  Transfer Fcn : TransferFcn  Numerator=1  Denominator=[tc 1]
  Voltage Sensor : fl_lib/Electrical/Electrical Sensors/Voltage Sensor
  neg : PMIOPort  Side=Right
  pos : PMIOPort  Port=2  Side=Left
  U : Outport
  wires:
  PS-Simulink Converter/1 -> Transfer Fcn/1
  Transfer Fcn/1 -> U/1
  connections:
  Voltage Sensor/RConn1 -- PS-Simulink Converter/LConn1
  Voltage Sensor/RConn2 -- neg/RConn1
  Voltage Sensor/LConn1 -- pos/RConn1

== stateflow chart Sim_Modell_v5/EM/Management Logic ==
  state normal_current
    entry:
    oc = 0;
  state over_current
    entry:
    oc = 1;
  (default) -> normal_current
  normal_current -> over_current : [Home_I >= 3]
  over_current -> normal_current : [Home_I < 3]
  data: Home_I input; oc output
